simulink model "tennode_3"  (R2018b)
settings: Solver=ode3  StartTime=0.0  StopTime=5  FixedStep=Ts  RelTol=1e-3
values from neighbouring files (symbols this model uses):
  BESS_mode = 0    [load_vars.m]
  line1 = line1_length*R1    (= 0.01273)    [load_vars.m]
  line10 = line10_length*R1    (= 0.01273)    [load_vars.m]
  LINE10_en = 1    [load_vars.m]
  line11 = line11_length*R1    (= 0.01273)    [load_vars.m]
  LINE11_en = 1    [load_vars.m]
  line12 = line12_length*R1    (= 0.02546)    [load_vars.m]
  LINE12_en = 1    [load_vars.m]
  line13 = line13_length*R1    (= 0.015276)    [load_vars.m]
  LINE13_en = 1    [load_vars.m]
  line14 = line14_length*R1    (= 0.019095)    [load_vars.m]
  LINE14_en = 1    [load_vars.m]
  line15 = line15_length*R1    (= 0.014003)    [load_vars.m]
  LINE15_en = 1    [load_vars.m]
  line16 = line16_length*R1    (= 0.034371)    [load_vars.m]
  LINE16_en = 1    [load_vars.m]
  line17 = line17_length*R1    (= 0.017822)    [load_vars.m]
  LINE17_en = 1    [load_vars.m]
  LINE1_en = 1    [load_vars.m]
  line2 = line2_length*R1    (= 0.02546)    [load_vars.m]
  LINE2_en = 1    [load_vars.m]
  line3 = line3_length*R1    (= 0.015276)    [load_vars.m]
  LINE3_en = 1    [load_vars.m]
  line4 = line4_length*R1    (= 0.019095)    [load_vars.m]
  LINE4_en = 1    [load_vars.m]
  line5 = line5_length*R1    (= 0.014003)    [load_vars.m]
  LINE5_en = 1    [load_vars.m]
  line6 = line6_length*R1    (= 0.01273)    [load_vars.m]
  LINE6_en = 1    [load_vars.m]
  line7 = line7_length*R1    (= 0.03819)    [load_vars.m]
  LINE7_en = 1    [load_vars.m]
  line8 = line8_length*R1    (= 0.01273)    [load_vars.m]
  LINE8_en = 1    [load_vars.m]
  line9 = line9_length*R1    (= 0.01273)    [load_vars.m]
  LINE9_en = 1    [load_vars.m]
  t_contingency = 1    [load_vars.m]
  Ts = 0.0001    [load_vars.m]
  uDemand1 = 20e3    (= 20000)    [load_vars.m]
  uDemand10 = 20e3    (= 20000)    [load_vars.m]
  uDemand2 = 20e3    (= 20000)    [load_vars.m]
  uDemand3 = 20e3    (= 20000)    [load_vars.m]
  uDemand4 = 20e3    (= 20000)    [load_vars.m]
  uDemand5 = 20e3    (= 20000)    [load_vars.m]
  uDemand6 = 20e3    (= 20000)    [load_vars.m]
  uDemand7 = 20e3    (= 20000)    [load_vars.m]
  uDemand8 = 20e3    (= 20000)    [load_vars.m]
  uDemand9 = 20e3    (= 20000)    [load_vars.m]
undefined symbols (not defined in the file or in its folder): DER10_BESS_en, DER1_BESS_en, DER2_BESS_en, DER3_BESS_en, DER4_BESS_en, DER5_BESS_en, DER6_BESS_en, DER7_BESS_en, DER8_BESS_en, DER9_BESS_en, DR_capacity_1, DR_capacity_10, DR_capacity_2, DR_capacity_3, DR_capacity_4, DR_capacity_5, DR_capacity_6, DR_capacity_7, DR_capacity_8, DR_capacity_9, P_set1, P_set10, P_set2, P_set3, P_set4, P_set5, P_set6, P_set7, P_set8, P_set9, PV_capacity_1, PV_capacity_10, PV_capacity_2, PV_capacity_3, PV_capacity_4, PV_capacity_5, PV_capacity_6, PV_capacity_7, PV_capacity_8, PV_capacity_9, PV_en_1, PV_en_10, PV_en_2, PV_en_3, PV_en_4, PV_en_5, PV_en_6, PV_en_7, PV_en_8, PV_en_9
libraries: powerlib x232, simulink x66, powerlib_meascontrol x23, sps_avr x1, spsDieselMotorModel x1
(part 6 of 7)

== system tennode_3/DER_Site_3/DER3_BESS/Stored Energy Calculation (%) ==
  Pin : Inport
  Qin : Inport  Port=2
  Charge : Gain  Gain=Efficiency/100
  Compare To Zero : simulink/Logic and Bit Operations/Compare To Zero  relop=<=  OutDataTypeStr=boolean
  Constant : Constant  Value=kWh_Rated
  Discharge : Gain  Gain=1/(Efficiency/100)
  Divide : Product  Inputs=*/
  Gain3 : Gain  Gain=1/3600/1e3
  Gain5 : Gain  Gain=-1
  Integrator : Integrator  InitialCondition=(Initial_kWh_pc/100)*kWh_Rated*3600*1e3
  Math Function1 : Math  Operator=square  SaturateOnIntegerOverflow=on
  Math Function2 : Math  Operator=square  SaturateOnIntegerOverflow=on
  Product : Product
  Sign : Signum
  Sqrt : Sqrt  SaturateOnIntegerOverflow=on
  Sum : Sum  Inputs=|++
  Switch1 : Switch  Criteria=u2 ~= 0
  Transfer Fcn : TransferFcn  Denominator=[1 1]
  to % : Gain  Gain=100
  SE% : Outport
  wires:
  Integrator/1 -> Gain3/1
  Compare To Zero/1 -> Switch1/2
  Divide/1 -> to %/1
  Charge/1 -> Switch1/1
  Constant/1 -> Divide/2
  Gain3/1 -> Divide/1
  Switch1/1 -> Gain5/1
  Transfer Fcn/1 -> Compare To Zero/1
  to %/1 -> SE%/1
  Gain5/1 -> Integrator/1
  Discharge/1 -> Switch1/3
  Product/1 -> Charge/1, Discharge/1, Transfer Fcn/1
  Pin/1 -> Sign/1, Math Function1/1
  Qin/1 -> Math Function2/1
  Math Function1/1 -> Sum/1
  Math Function2/1 -> Sum/2
  Sum/1 -> Sqrt/1
  Sqrt/1 -> Product/2
  Sign/1 -> Product/1

== system tennode_3/DER_Site_3/Site Load/Dynamic Load Control ==
  P0 : Inport
  Fcn : Fcn  Expr=sqrt(1/u(1)-1)
  Mux : Mux  Inputs=2
  Product : Product
  Summer1 : Constant  Value=PF
  PQ : Outport
  wires:
  Summer1/1 -> Fcn/1
  Fcn/1 -> Product/2
  P0/1 -> Product/1, Mux/1
  Mux/1 -> PQ/1
  Product/1 -> Mux/2  "Qo"

== system tennode_3/DER_Site_4/DER3_BESS1/Charge Limits ==
  SOC (%) : Inport
  Pin : Inport  Port=2
  Qin : Inport  Port=3
  Overcharge Check : Subsystem
  Undercharge Check : Subsystem
  Pbatt : Outport
  Qbatt : Outport  Port=2
  wires:
  Overcharge Check/2(Qout) -> Undercharge Check/3(Qin)
  Undercharge Check/1(Pout) -> Pbatt/1  "Pbatt"
  Qin/1 -> Overcharge Check/3(Qin)
  Overcharge Check/1(Pout) -> Undercharge Check/2(Pin)
  Pin/1 -> Overcharge Check/2(Pin)
  Undercharge Check/2(Qout) -> Qbatt/1
  SOC (%)/1 -> Undercharge Check/1(SOC (%)), Overcharge Check/1(SOC (%))

== system tennode_3/DER_Site_4/DER3_BESS1/Disable PQ Source if VF Control ==
  Pdes : Inport
  Mode : Inport  Port=2
  Qdes : Inport  Port=3
  Constant : Constant  Value=0
  Constant1 : Constant  Value=0
  Switch2 : Switch  Criteria=u2 > Threshold
  Switch3 : Switch  Criteria=u2 > Threshold
  Pbatt : Outport
  Qbatt : Outport  Port=2
  wires:
  Qdes/1 -> Switch3/1
  Constant/1 -> Switch2/3
  Switch3/1 -> Qbatt/1
  Constant1/1 -> Switch3/3
  Switch2/1 -> Pbatt/1
  Pdes/1 -> Switch2/1
  Mode/1 -> Switch2/2, Switch3/2

== system tennode_3/DER_Site_4/DER3_BESS1/Power Measures ==
  EMT : Subsystem  VariantControl=EMT
  Phasor : Subsystem  VariantControl=Phasor
  A : PMIOPort  Side=Left
  a : PMIOPort  Port=2  Side=Right
  B : PMIOPort  Port=3  Side=Left
  b : PMIOPort  Port=4  Side=Right
  C : PMIOPort  Port=5  Side=Left
  c : PMIOPort  Port=6  Side=Right
  P : Outport
  Q : Outport  Port=2

== system tennode_3/DER_Site_4/DER3_BESS1/Reactive Power Capability ==
  Pin : Inport
  Qin : Inport  Port=2
  Constant : Constant  Value=Pnom
  Math Function : Math  Operator=square  SaturateOnIntegerOverflow=on
  Math Function1 : Math  Operator=square  SaturateOnIntegerOverflow=on
  Saturation Dynamic : simulink/Discontinuities/Saturation Dynamic  OutMin=[]  OutMax=[]  OutDataTypeStr=Inherit: Same as second input  OutDataType=fixdt(1, 16)  OutScaling=2^-10  DoSatur=off
  Sqrt : Sqrt  SaturateOnIntegerOverflow=on
  Sum : Sum  Inputs=-+|
  Unary Minus : UnaryMinus
  Qout : Outport
  wires:
  Qin/1 -> Saturation Dynamic/2
  Pin/1 -> Math Function1/1
  Saturation Dynamic/1 -> Qout/1
  Unary Minus/1 -> Saturation Dynamic/3
  Sum/1 -> Sqrt/1
  Constant/1 -> Math Function/1
  Math Function/1 -> Sum/2
  Math Function1/1 -> Sum/1
  Sqrt/1 -> Unary Minus/1, Saturation Dynamic/1

== system tennode_3/DER_Site_4/DER3_BESS1/Stored Energy Calculation (%) ==
  Pin : Inport
  Qin : Inport  Port=2
  Charge : Gain  Gain=Efficiency/100
  Compare To Zero : simulink/Logic and Bit Operations/Compare To Zero  relop=<=  OutDataTypeStr=boolean
  Constant : Constant  Value=kWh_Rated
  Discharge : Gain  Gain=1/(Efficiency/100)
  Divide : Product  Inputs=*/
  Gain3 : Gain  Gain=1/3600/1e3
  Gain5 : Gain  Gain=-1
  Integrator : Integrator  InitialCondition=(Initial_kWh_pc/100)*kWh_Rated*3600*1e3
  Math Function1 : Math  Operator=square  SaturateOnIntegerOverflow=on
  Math Function2 : Math  Operator=square  SaturateOnIntegerOverflow=on
  Product : Product
  Sign : Signum
  Sqrt : Sqrt  SaturateOnIntegerOverflow=on
  Sum : Sum  Inputs=|++
  Switch1 : Switch  Criteria=u2 ~= 0
  Transfer Fcn : TransferFcn  Denominator=[1 1]
  to % : Gain  Gain=100
  SE% : Outport
  wires:
  Integrator/1 -> Gain3/1
  Compare To Zero/1 -> Switch1/2
  Divide/1 -> to %/1
  Charge/1 -> Switch1/1
  Constant/1 -> Divide/2
  Gain3/1 -> Divide/1
  Switch1/1 -> Gain5/1
  Transfer Fcn/1 -> Compare To Zero/1
  to %/1 -> SE%/1
  Gain5/1 -> Integrator/1
  Discharge/1 -> Switch1/3
  Product/1 -> Charge/1, Discharge/1, Transfer Fcn/1
  Pin/1 -> Sign/1, Math Function1/1
  Qin/1 -> Math Function2/1
  Math Function1/1 -> Sum/1
  Math Function2/1 -> Sum/2
  Sum/1 -> Sqrt/1
  Sqrt/1 -> Product/2
  Sign/1 -> Product/1

== system tennode_3/DER_Site_4/Site Load/Dynamic Load Control ==
  P0 : Inport
  Fcn : Fcn  Expr=sqrt(1/u(1)-1)
  Mux : Mux  Inputs=2
  Product : Product
  Summer1 : Constant  Value=PF
  PQ : Outport
  wires:
  Summer1/1 -> Fcn/1
  Fcn/1 -> Product/2
  P0/1 -> Product/1, Mux/1
  Mux/1 -> PQ/1
  Product/1 -> Mux/2  "Qo"

== system tennode_3/DER_Site_5/DER3_BESS1/Charge Limits ==
  SOC (%) : Inport
  Pin : Inport  Port=2
  Qin : Inport  Port=3
  Overcharge Check : Subsystem
  Undercharge Check : Subsystem
  Pbatt : Outport
  Qbatt : Outport  Port=2
  wires:
  Overcharge Check/2(Qout) -> Undercharge Check/3(Qin)
  Undercharge Check/1(Pout) -> Pbatt/1  "Pbatt"
  Qin/1 -> Overcharge Check/3(Qin)
  Overcharge Check/1(Pout) -> Undercharge Check/2(Pin)
  Pin/1 -> Overcharge Check/2(Pin)
  Undercharge Check/2(Qout) -> Qbatt/1
  SOC (%)/1 -> Undercharge Check/1(SOC (%)), Overcharge Check/1(SOC (%))

== system tennode_3/DER_Site_5/DER3_BESS1/Disable PQ Source if VF Control ==
  Pdes : Inport
  Mode : Inport  Port=2
  Qdes : Inport  Port=3
  Constant : Constant  Value=0
  Constant1 : Constant  Value=0
  Switch2 : Switch  Criteria=u2 > Threshold
  Switch3 : Switch  Criteria=u2 > Threshold
  Pbatt : Outport
  Qbatt : Outport  Port=2
  wires:
  Qdes/1 -> Switch3/1
  Constant/1 -> Switch2/3
  Switch3/1 -> Qbatt/1
  Constant1/1 -> Switch3/3
  Switch2/1 -> Pbatt/1
  Pdes/1 -> Switch2/1
  Mode/1 -> Switch2/2, Switch3/2

== system tennode_3/DER_Site_5/DER3_BESS1/Power Measures ==
  EMT : Subsystem  VariantControl=EMT
  Phasor : Subsystem  VariantControl=Phasor
  A : PMIOPort  Side=Left
  a : PMIOPort  Port=2  Side=Right
  B : PMIOPort  Port=3  Side=Left
  b : PMIOPort  Port=4  Side=Right
  C : PMIOPort  Port=5  Side=Left
  c : PMIOPort  Port=6  Side=Right
  P : Outport
  Q : Outport  Port=2

== system tennode_3/DER_Site_5/DER3_BESS1/Reactive Power Capability ==
  Pin : Inport
  Qin : Inport  Port=2
  Constant : Constant  Value=Pnom
  Math Function : Math  Operator=square  SaturateOnIntegerOverflow=on
  Math Function1 : Math  Operator=square  SaturateOnIntegerOverflow=on
  Saturation Dynamic : simulink/Discontinuities/Saturation Dynamic  OutMin=[]  OutMax=[]  OutDataTypeStr=Inherit: Same as second input  OutDataType=fixdt(1, 16)  OutScaling=2^-10  DoSatur=off
  Sqrt : Sqrt  SaturateOnIntegerOverflow=on
  Sum : Sum  Inputs=-+|
  Unary Minus : UnaryMinus
  Qout : Outport
  wires:
  Qin/1 -> Saturation Dynamic/2
  Pin/1 -> Math Function1/1
  Saturation Dynamic/1 -> Qout/1
  Unary Minus/1 -> Saturation Dynamic/3
  Sum/1 -> Sqrt/1
  Constant/1 -> Math Function/1
  Math Function/1 -> Sum/2
  Math Function1/1 -> Sum/1
  Sqrt/1 -> Unary Minus/1, Saturation Dynamic/1

== system tennode_3/DER_Site_5/DER3_BESS1/Stored Energy Calculation (%) ==
  Pin : Inport
  Qin : Inport  Port=2
  Charge : Gain  Gain=Efficiency/100
  Compare To Zero : simulink/Logic and Bit Operations/Compare To Zero  relop=<=  OutDataTypeStr=boolean
  Constant : Constant  Value=kWh_Rated
  Discharge : Gain  Gain=1/(Efficiency/100)
  Divide : Product  Inputs=*/
  Gain3 : Gain  Gain=1/3600/1e3
  Gain5 : Gain  Gain=-1
  Integrator : Integrator  InitialCondition=(Initial_kWh_pc/100)*kWh_Rated*3600*1e3
  Math Function1 : Math  Operator=square  SaturateOnIntegerOverflow=on
  Math Function2 : Math  Operator=square  SaturateOnIntegerOverflow=on
  Product : Product
  Sign : Signum
  Sqrt : Sqrt  SaturateOnIntegerOverflow=on
  Sum : Sum  Inputs=|++
  Switch1 : Switch  Criteria=u2 ~= 0
  Transfer Fcn : TransferFcn  Denominator=[1 1]
  to % : Gain  Gain=100
  SE% : Outport
  wires:
  Integrator/1 -> Gain3/1
  Compare To Zero/1 -> Switch1/2
  Divide/1 -> to %/1
  Charge/1 -> Switch1/1
  Constant/1 -> Divide/2
  Gain3/1 -> Divide/1
  Switch1/1 -> Gain5/1
  Transfer Fcn/1 -> Compare To Zero/1
  to %/1 -> SE%/1
  Gain5/1 -> Integrator/1
  Discharge/1 -> Switch1/3
  Product/1 -> Charge/1, Discharge/1, Transfer Fcn/1
  Pin/1 -> Sign/1, Math Function1/1
  Qin/1 -> Math Function2/1
  Math Function1/1 -> Sum/1
  Math Function2/1 -> Sum/2
  Sum/1 -> Sqrt/1
  Sqrt/1 -> Product/2
  Sign/1 -> Product/1

== system tennode_3/DER_Site_5/Site Load/Dynamic Load Control ==
  P0 : Inport
  Fcn : Fcn  Expr=sqrt(1/u(1)-1)
  Mux : Mux  Inputs=2
  Product : Product
  Summer1 : Constant  Value=PF
  PQ : Outport
  wires:
  Summer1/1 -> Fcn/1
  Fcn/1 -> Product/2
  P0/1 -> Product/1, Mux/1
  Mux/1 -> PQ/1
  Product/1 -> Mux/2  "Qo"

== system tennode_3/DER_Site_6/DER6_BESS/Charge Limits ==
  SOC (%) : Inport
  Pin : Inport  Port=2
  Qin : Inport  Port=3
  Overcharge Check : Subsystem
  Undercharge Check : Subsystem
  Pbatt : Outport
  Qbatt : Outport  Port=2
  wires:
  Overcharge Check/2(Qout) -> Undercharge Check/3(Qin)
  Undercharge Check/1(Pout) -> Pbatt/1  "Pbatt"
  Qin/1 -> Overcharge Check/3(Qin)
  Overcharge Check/1(Pout) -> Undercharge Check/2(Pin)
  Pin/1 -> Overcharge Check/2(Pin)
  Undercharge Check/2(Qout) -> Qbatt/1
  SOC (%)/1 -> Undercharge Check/1(SOC (%)), Overcharge Check/1(SOC (%))

== system tennode_3/DER_Site_6/DER6_BESS/Disable PQ Source if VF Control ==
  Pdes : Inport
  Mode : Inport  Port=2
  Qdes : Inport  Port=3
  Constant : Constant  Value=0
  Constant1 : Constant  Value=0
  Switch2 : Switch  Criteria=u2 > Threshold
  Switch3 : Switch  Criteria=u2 > Threshold
  Pbatt : Outport
  Qbatt : Outport  Port=2
  wires:
  Qdes/1 -> Switch3/1
  Constant/1 -> Switch2/3
  Switch3/1 -> Qbatt/1
  Constant1/1 -> Switch3/3
  Switch2/1 -> Pbatt/1
  Pdes/1 -> Switch2/1
  Mode/1 -> Switch2/2, Switch3/2

== system tennode_3/DER_Site_6/DER6_BESS/Power Measures ==
  EMT : Subsystem  VariantControl=EMT
  Phasor : Subsystem  VariantControl=Phasor
  A : PMIOPort  Side=Left
  a : PMIOPort  Port=2  Side=Right
  B : PMIOPort  Port=3  Side=Left
  b : PMIOPort  Port=4  Side=Right
  C : PMIOPort  Port=5  Side=Left
  c : PMIOPort  Port=6  Side=Right
  P : Outport
  Q : Outport  Port=2

== system tennode_3/DER_Site_6/DER6_BESS/Reactive Power Capability ==
  Pin : Inport
  Qin : Inport  Port=2
  Constant : Constant  Value=Pnom
  Math Function : Math  Operator=square  SaturateOnIntegerOverflow=on
  Math Function1 : Math  Operator=square  SaturateOnIntegerOverflow=on
  Saturation Dynamic : simulink/Discontinuities/Saturation Dynamic  OutMin=[]  OutMax=[]  OutDataTypeStr=Inherit: Same as second input  OutDataType=fixdt(1, 16)  OutScaling=2^-10  DoSatur=off
  Sqrt : Sqrt  SaturateOnIntegerOverflow=on
  Sum : Sum  Inputs=-+|
  Unary Minus : UnaryMinus
  Qout : Outport
  wires:
  Qin/1 -> Saturation Dynamic/2
  Pin/1 -> Math Function1/1
  Saturation Dynamic/1 -> Qout/1
  Unary Minus/1 -> Saturation Dynamic/3
  Sum/1 -> Sqrt/1
  Constant/1 -> Math Function/1
  Math Function/1 -> Sum/2
  Math Function1/1 -> Sum/1
  Sqrt/1 -> Unary Minus/1, Saturation Dynamic/1

== system tennode_3/DER_Site_6/DER6_BESS/Stored Energy Calculation (%) ==
  Pin : Inport
  Qin : Inport  Port=2
  Charge : Gain  Gain=Efficiency/100
  Compare To Zero : simulink/Logic and Bit Operations/Compare To Zero  relop=<=  OutDataTypeStr=boolean
  Constant : Constant  Value=kWh_Rated
  Discharge : Gain  Gain=1/(Efficiency/100)
  Divide : Product  Inputs=*/
  Gain3 : Gain  Gain=1/3600/1e3
  Gain5 : Gain  Gain=-1
  Integrator : Integrator  InitialCondition=(Initial_kWh_pc/100)*kWh_Rated*3600*1e3
  Math Function1 : Math  Operator=square  SaturateOnIntegerOverflow=on
  Math Function2 : Math  Operator=square  SaturateOnIntegerOverflow=on
  Product : Product
  Sign : Signum
  Sqrt : Sqrt  SaturateOnIntegerOverflow=on
  Sum : Sum  Inputs=|++
  Switch1 : Switch  Criteria=u2 ~= 0
  Transfer Fcn : TransferFcn  Denominator=[1 1]
  to % : Gain  Gain=100
  SE% : Outport
  wires:
  Integrator/1 -> Gain3/1
  Compare To Zero/1 -> Switch1/2
  Divide/1 -> to %/1
  Charge/1 -> Switch1/1
  Constant/1 -> Divide/2
  Gain3/1 -> Divide/1
  Switch1/1 -> Gain5/1
  Transfer Fcn/1 -> Compare To Zero/1
  to %/1 -> SE%/1
  Gain5/1 -> Integrator/1
  Discharge/1 -> Switch1/3
  Product/1 -> Charge/1, Discharge/1, Transfer Fcn/1
  Pin/1 -> Sign/1, Math Function1/1
  Qin/1 -> Math Function2/1
  Math Function1/1 -> Sum/1
  Math Function2/1 -> Sum/2
  Sum/1 -> Sqrt/1
  Sqrt/1 -> Product/2
  Sign/1 -> Product/1

== system tennode_3/DER_Site_6/Site Load/Dynamic Load Control ==
  P0 : Inport
  Fcn : Fcn  Expr=sqrt(1/u(1)-1)
  Mux : Mux  Inputs=2
  Product : Product
  Summer1 : Constant  Value=PF
  PQ : Outport
  wires:
  Summer1/1 -> Fcn/1
  Fcn/1 -> Product/2
  P0/1 -> Product/1, Mux/1
  Mux/1 -> PQ/1
  Product/1 -> Mux/2  "Qo"

== system tennode_3/DER_Site_7/DER7_BESS/Charge Limits ==
  SOC (%) : Inport
  Pin : Inport  Port=2
  Qin : Inport  Port=3
  Overcharge Check : Subsystem
  Undercharge Check : Subsystem
  Pbatt : Outport
  Qbatt : Outport  Port=2
  wires:
  Overcharge Check/2(Qout) -> Undercharge Check/3(Qin)
  Undercharge Check/1(Pout) -> Pbatt/1  "Pbatt"
  Qin/1 -> Overcharge Check/3(Qin)
  Overcharge Check/1(Pout) -> Undercharge Check/2(Pin)
  Pin/1 -> Overcharge Check/2(Pin)
  Undercharge Check/2(Qout) -> Qbatt/1
  SOC (%)/1 -> Undercharge Check/1(SOC (%)), Overcharge Check/1(SOC (%))

== system tennode_3/DER_Site_7/DER7_BESS/Disable PQ Source if VF Control ==
  Pdes : Inport
  Mode : Inport  Port=2
  Qdes : Inport  Port=3
  Constant : Constant  Value=0
  Constant1 : Constant  Value=0
  Switch2 : Switch  Criteria=u2 > Threshold
  Switch3 : Switch  Criteria=u2 > Threshold
  Pbatt : Outport
  Qbatt : Outport  Port=2
  wires:
  Qdes/1 -> Switch3/1
  Constant/1 -> Switch2/3
  Switch3/1 -> Qbatt/1
  Constant1/1 -> Switch3/3
  Switch2/1 -> Pbatt/1
  Pdes/1 -> Switch2/1
  Mode/1 -> Switch2/2, Switch3/2

== system tennode_3/DER_Site_7/DER7_BESS/Power Measures ==
  EMT : Subsystem  VariantControl=EMT
  Phasor : Subsystem  VariantControl=Phasor
  A : PMIOPort  Side=Left
  a : PMIOPort  Port=2  Side=Right
  B : PMIOPort  Port=3  Side=Left
  b : PMIOPort  Port=4  Side=Right
  C : PMIOPort  Port=5  Side=Left
  c : PMIOPort  Port=6  Side=Right
  P : Outport
  Q : Outport  Port=2

== system tennode_3/DER_Site_7/DER7_BESS/Reactive Power Capability ==
  Pin : Inport
  Qin : Inport  Port=2
  Constant : Constant  Value=Pnom
  Math Function : Math  Operator=square  SaturateOnIntegerOverflow=on
  Math Function1 : Math  Operator=square  SaturateOnIntegerOverflow=on
  Saturation Dynamic : simulink/Discontinuities/Saturation Dynamic  OutMin=[]  OutMax=[]  OutDataTypeStr=Inherit: Same as second input  OutDataType=fixdt(1, 16)  OutScaling=2^-10  DoSatur=off
  Sqrt : Sqrt  SaturateOnIntegerOverflow=on
  Sum : Sum  Inputs=-+|
  Unary Minus : UnaryMinus
  Qout : Outport
  wires:
  Qin/1 -> Saturation Dynamic/2
  Pin/1 -> Math Function1/1
  Saturation Dynamic/1 -> Qout/1
  Unary Minus/1 -> Saturation Dynamic/3
  Sum/1 -> Sqrt/1
  Constant/1 -> Math Function/1
  Math Function/1 -> Sum/2
  Math Function1/1 -> Sum/1
  Sqrt/1 -> Unary Minus/1, Saturation Dynamic/1

== system tennode_3/DER_Site_7/DER7_BESS/Stored Energy Calculation (%) ==
  Pin : Inport
  Qin : Inport  Port=2
  Charge : Gain  Gain=Efficiency/100
  Compare To Zero : simulink/Logic and Bit Operations/Compare To Zero  relop=<=  OutDataTypeStr=boolean
  Constant : Constant  Value=kWh_Rated
  Discharge : Gain  Gain=1/(Efficiency/100)
  Divide : Product  Inputs=*/
  Gain3 : Gain  Gain=1/3600/1e3
  Gain5 : Gain  Gain=-1
  Integrator : Integrator  InitialCondition=(Initial_kWh_pc/100)*kWh_Rated*3600*1e3
  Math Function1 : Math  Operator=square  SaturateOnIntegerOverflow=on
  Math Function2 : Math  Operator=square  SaturateOnIntegerOverflow=on
  Product : Product
  Sign : Signum
  Sqrt : Sqrt  SaturateOnIntegerOverflow=on
  Sum : Sum  Inputs=|++
  Switch1 : Switch  Criteria=u2 ~= 0
  Transfer Fcn : TransferFcn  Denominator=[1 1]
  to % : Gain  Gain=100
  SE% : Outport
  wires:
  Integrator/1 -> Gain3/1
  Compare To Zero/1 -> Switch1/2
  Divide/1 -> to %/1
  Charge/1 -> Switch1/1
  Constant/1 -> Divide/2
  Gain3/1 -> Divide/1
  Switch1/1 -> Gain5/1
  Transfer Fcn/1 -> Compare To Zero/1
  to %/1 -> SE%/1
  Gain5/1 -> Integrator/1
  Discharge/1 -> Switch1/3
  Product/1 -> Charge/1, Discharge/1, Transfer Fcn/1
  Pin/1 -> Sign/1, Math Function1/1
  Qin/1 -> Math Function2/1
  Math Function1/1 -> Sum/1
  Math Function2/1 -> Sum/2
  Sum/1 -> Sqrt/1
  Sqrt/1 -> Product/2
  Sign/1 -> Product/1

== system tennode_3/DER_Site_7/Site Load/Dynamic Load Control ==
  P0 : Inport
  Fcn : Fcn  Expr=sqrt(1/u(1)-1)
  Mux : Mux  Inputs=2
  Product : Product
  Summer1 : Constant  Value=PF
  PQ : Outport
  wires:
  Summer1/1 -> Fcn/1
  Fcn/1 -> Product/2
  P0/1 -> Product/1, Mux/1
  Mux/1 -> PQ/1
  Product/1 -> Mux/2  "Qo"

== system tennode_3/DER_Site_8/DER8_BESS/Charge Limits ==
  SOC (%) : Inport
  Pin : Inport  Port=2
  Qin : Inport  Port=3
  Overcharge Check : Subsystem
  Undercharge Check : Subsystem
  Pbatt : Outport
  Qbatt : Outport  Port=2
  wires:
  Overcharge Check/2(Qout) -> Undercharge Check/3(Qin)
  Undercharge Check/1(Pout) -> Pbatt/1  "Pbatt"
  Qin/1 -> Overcharge Check/3(Qin)
  Overcharge Check/1(Pout) -> Undercharge Check/2(Pin)
  Pin/1 -> Overcharge Check/2(Pin)
  Undercharge Check/2(Qout) -> Qbatt/1
  SOC (%)/1 -> Undercharge Check/1(SOC (%)), Overcharge Check/1(SOC (%))

== system tennode_3/DER_Site_8/DER8_BESS/Disable PQ Source if VF Control ==
  Pdes : Inport
  Mode : Inport  Port=2
  Qdes : Inport  Port=3
  Constant : Constant  Value=0
  Constant1 : Constant  Value=0
  Switch2 : Switch  Criteria=u2 > Threshold
  Switch3 : Switch  Criteria=u2 > Threshold
  Pbatt : Outport
  Qbatt : Outport  Port=2
  wires:
  Qdes/1 -> Switch3/1
  Constant/1 -> Switch2/3
  Switch3/1 -> Qbatt/1
  Constant1/1 -> Switch3/3
  Switch2/1 -> Pbatt/1
  Pdes/1 -> Switch2/1
  Mode/1 -> Switch2/2, Switch3/2

== system tennode_3/DER_Site_8/DER8_BESS/Power Measures ==
  EMT : Subsystem  VariantControl=EMT
  Phasor : Subsystem  VariantControl=Phasor
  A : PMIOPort  Side=Left
  a : PMIOPort  Port=2  Side=Right
  B : PMIOPort  Port=3  Side=Left
  b : PMIOPort  Port=4  Side=Right
  C : PMIOPort  Port=5  Side=Left
  c : PMIOPort  Port=6  Side=Right
  P : Outport
  Q : Outport  Port=2

== system tennode_3/DER_Site_8/DER8_BESS/Reactive Power Capability ==
  Pin : Inport
  Qin : Inport  Port=2
  Constant : Constant  Value=Pnom
  Math Function : Math  Operator=square  SaturateOnIntegerOverflow=on
  Math Function1 : Math  Operator=square  SaturateOnIntegerOverflow=on
  Saturation Dynamic : simulink/Discontinuities/Saturation Dynamic  OutMin=[]  OutMax=[]  OutDataTypeStr=Inherit: Same as second input  OutDataType=fixdt(1, 16)  OutScaling=2^-10  DoSatur=off
  Sqrt : Sqrt  SaturateOnIntegerOverflow=on
  Sum : Sum  Inputs=-+|
  Unary Minus : UnaryMinus
  Qout : Outport
  wires:
  Qin/1 -> Saturation Dynamic/2
  Pin/1 -> Math Function1/1
  Saturation Dynamic/1 -> Qout/1
  Unary Minus/1 -> Saturation Dynamic/3
  Sum/1 -> Sqrt/1
  Constant/1 -> Math Function/1
  Math Function/1 -> Sum/2
  Math Function1/1 -> Sum/1
  Sqrt/1 -> Unary Minus/1, Saturation Dynamic/1

== system tennode_3/DER_Site_8/DER8_BESS/Stored Energy Calculation (%) ==
  Pin : Inport
  Qin : Inport  Port=2
  Charge : Gain  Gain=Efficiency/100
  Compare To Zero : simulink/Logic and Bit Operations/Compare To Zero  relop=<=  OutDataTypeStr=boolean
  Constant : Constant  Value=kWh_Rated
  Discharge : Gain  Gain=1/(Efficiency/100)
  Divide : Product  Inputs=*/
  Gain3 : Gain  Gain=1/3600/1e3
  Gain5 : Gain  Gain=-1
  Integrator : Integrator  InitialCondition=(Initial_kWh_pc/100)*kWh_Rated*3600*1e3
  Math Function1 : Math  Operator=square  SaturateOnIntegerOverflow=on
  Math Function2 : Math  Operator=square  SaturateOnIntegerOverflow=on
  Product : Product
  Sign : Signum
  Sqrt : Sqrt  SaturateOnIntegerOverflow=on
  Sum : Sum  Inputs=|++
  Switch1 : Switch  Criteria=u2 ~= 0
  Transfer Fcn : TransferFcn  Denominator=[1 1]
  to % : Gain  Gain=100
  SE% : Outport
  wires:
  Integrator/1 -> Gain3/1
  Compare To Zero/1 -> Switch1/2
  Divide/1 -> to %/1
  Charge/1 -> Switch1/1
  Constant/1 -> Divide/2
  Gain3/1 -> Divide/1
  Switch1/1 -> Gain5/1
  Transfer Fcn/1 -> Compare To Zero/1
  to %/1 -> SE%/1
  Gain5/1 -> Integrator/1
  Discharge/1 -> Switch1/3
  Product/1 -> Charge/1, Discharge/1, Transfer Fcn/1
  Pin/1 -> Sign/1, Math Function1/1
  Qin/1 -> Math Function2/1
  Math Function1/1 -> Sum/1
  Math Function2/1 -> Sum/2
  Sum/1 -> Sqrt/1
  Sqrt/1 -> Product/2
  Sign/1 -> Product/1

== system tennode_3/DER_Site_8/Site Load/Dynamic Load Control ==
  P0 : Inport
  Fcn : Fcn  Expr=sqrt(1/u(1)-1)
  Mux : Mux  Inputs=2
  Product : Product
  Summer1 : Constant  Value=PF
  PQ : Outport
  wires:
  Summer1/1 -> Fcn/1
  Fcn/1 -> Product/2
  P0/1 -> Product/1, Mux/1
  Mux/1 -> PQ/1
  Product/1 -> Mux/2  "Qo"

== system tennode_3/DER_Site_9/DER9_BESS/Charge Limits ==
  SOC (%) : Inport
  Pin : Inport  Port=2
  Qin : Inport  Port=3
  Overcharge Check : Subsystem
  Undercharge Check : Subsystem
  Pbatt : Outport
  Qbatt : Outport  Port=2
  wires:
  Overcharge Check/2(Qout) -> Undercharge Check/3(Qin)
  Undercharge Check/1(Pout) -> Pbatt/1  "Pbatt"
  Qin/1 -> Overcharge Check/3(Qin)
  Overcharge Check/1(Pout) -> Undercharge Check/2(Pin)
  Pin/1 -> Overcharge Check/2(Pin)
  Undercharge Check/2(Qout) -> Qbatt/1
  SOC (%)/1 -> Undercharge Check/1(SOC (%)), Overcharge Check/1(SOC (%))

== system tennode_3/DER_Site_9/DER9_BESS/Disable PQ Source if VF Control ==
  Pdes : Inport
  Mode : Inport  Port=2
  Qdes : Inport  Port=3
  Constant : Constant  Value=0
  Constant1 : Constant  Value=0
  Switch2 : Switch  Criteria=u2 > Threshold
  Switch3 : Switch  Criteria=u2 > Threshold
  Pbatt : Outport
  Qbatt : Outport  Port=2
  wires:
  Qdes/1 -> Switch3/1
  Constant/1 -> Switch2/3
  Switch3/1 -> Qbatt/1
  Constant1/1 -> Switch3/3
  Switch2/1 -> Pbatt/1
  Pdes/1 -> Switch2/1
  Mode/1 -> Switch2/2, Switch3/2

== system tennode_3/DER_Site_9/DER9_BESS/Power Measures ==
  EMT : Subsystem  VariantControl=EMT
  Phasor : Subsystem  VariantControl=Phasor
  A : PMIOPort  Side=Left
  a : PMIOPort  Port=2  Side=Right
  B : PMIOPort  Port=3  Side=Left
  b : PMIOPort  Port=4  Side=Right
  C : PMIOPort  Port=5  Side=Left
  c : PMIOPort  Port=6  Side=Right
  P : Outport
  Q : Outport  Port=2

== system tennode_3/DER_Site_9/DER9_BESS/Reactive Power Capability ==
  Pin : Inport
  Qin : Inport  Port=2
  Constant : Constant  Value=Pnom
  Math Function : Math  Operator=square  SaturateOnIntegerOverflow=on
  Math Function1 : Math  Operator=square  SaturateOnIntegerOverflow=on
  Saturation Dynamic : simulink/Discontinuities/Saturation Dynamic  OutMin=[]  OutMax=[]  OutDataTypeStr=Inherit: Same as second input  OutDataType=fixdt(1, 16)  OutScaling=2^-10  DoSatur=off
  Sqrt : Sqrt  SaturateOnIntegerOverflow=on
  Sum : Sum  Inputs=-+|
  Unary Minus : UnaryMinus
  Qout : Outport
  wires:
  Qin/1 -> Saturation Dynamic/2
  Pin/1 -> Math Function1/1
  Saturation Dynamic/1 -> Qout/1
  Unary Minus/1 -> Saturation Dynamic/3
  Sum/1 -> Sqrt/1
  Constant/1 -> Math Function/1
  Math Function/1 -> Sum/2
  Math Function1/1 -> Sum/1
  Sqrt/1 -> Unary Minus/1, Saturation Dynamic/1

== system tennode_3/DER_Site_9/DER9_BESS/Stored Energy Calculation (%) ==
  Pin : Inport
  Qin : Inport  Port=2
  Charge : Gain  Gain=Efficiency/100
  Compare To Zero : simulink/Logic and Bit Operations/Compare To Zero  relop=<=  OutDataTypeStr=boolean
  Constant : Constant  Value=kWh_Rated
  Discharge : Gain  Gain=1/(Efficiency/100)
  Divide : Product  Inputs=*/
  Gain3 : Gain  Gain=1/3600/1e3
  Gain5 : Gain  Gain=-1
  Integrator : Integrator  InitialCondition=(Initial_kWh_pc/100)*kWh_Rated*3600*1e3
  Math Function1 : Math  Operator=square  SaturateOnIntegerOverflow=on
  Math Function2 : Math  Operator=square  SaturateOnIntegerOverflow=on
  Product : Product
  Sign : Signum
  Sqrt : Sqrt  SaturateOnIntegerOverflow=on
  Sum : Sum  Inputs=|++
  Switch1 : Switch  Criteria=u2 ~= 0
  Transfer Fcn : TransferFcn  Denominator=[1 1]
  to % : Gain  Gain=100
  SE% : Outport
  wires:
  Integrator/1 -> Gain3/1
  Compare To Zero/1 -> Switch1/2
  Divide/1 -> to %/1
  Charge/1 -> Switch1/1
  Constant/1 -> Divide/2
  Gain3/1 -> Divide/1
  Switch1/1 -> Gain5/1
  Transfer Fcn/1 -> Compare To Zero/1
  to %/1 -> SE%/1
  Gain5/1 -> Integrator/1
  Discharge/1 -> Switch1/3
  Product/1 -> Charge/1, Discharge/1, Transfer Fcn/1
  Pin/1 -> Sign/1, Math Function1/1
  Qin/1 -> Math Function2/1
  Math Function1/1 -> Sum/1
  Math Function2/1 -> Sum/2
  Sum/1 -> Sqrt/1
  Sqrt/1 -> Product/2
  Sign/1 -> Product/1

== system tennode_3/DER_Site_9/Site Load/Dynamic Load Control ==
  P0 : Inport
  Fcn : Fcn  Expr=sqrt(1/u(1)-1)
  Mux : Mux  Inputs=2
  Product : Product
  Summer1 : Constant  Value=PF
  PQ : Outport
  wires:
  Summer1/1 -> Fcn/1
  Fcn/1 -> Product/2
  P0/1 -> Product/1, Mux/1
  Mux/1 -> PQ/1
  Product/1 -> Mux/2  "Qo"

== system tennode_3/Frequency Measure/Diesel Generator/Generator Measures ==
  m : Inport
  Bus Selector : BusSelector  OutputSignals="dq0 components.Stator voltage  vq (pu),dq0 components.Stator voltage  vd (pu)"  OutputAsBus=on
  Bus Selector1 : BusSelector  OutputSignals="Mechanical.Rotor speed  wm  (pu),dq0 components.Field current  ifd (pu)"
  Fcn1 : Fcn  Expr=sqrt(u(1)^2 + u(2)^2)
  Ifd : Outport
  Vt : Outport  Port=2
  wm : Outport  Port=3
  wires:
  Bus Selector1/1 -> wm/1  "<Rotor speed  wm  (pu)>"
  m/1 -> Bus Selector1/1, Bus Selector/1
  Fcn1/1 -> Vt/1
  Bus Selector/1 -> Fcn1/1
  Bus Selector1/2 -> Ifd/1  "<Field current  ifd (pu)>"

== system tennode_3/Frequency Measure/Diesel Generator/Selected Measurements ==
  m : Inport
  Bus Creator : BusCreator  Inputs=7
  Bus Selector : BusSelector  OutputSignals="Mechanical.Electrical power  Pe (pu),Mechanical.Rotor speed  wm  (pu),Output active power   Peo (pu),Output reactive power  Qeo (pu)"
  to W : Gain  Gain=Pn
  to W1 : Gain  Gain=Pn
  to W2 : Gain  Gain=Pn
  sm : Outport
  wires:
  to W2/1 -> Bus Creator/7  "Reactive Power (W)"
  to W1/1 -> Bus Creator/6  "Active Power (W)"
  Bus Selector/2 -> Bus Creator/3  "<Rotor speed  wm  (pu)>"
  Bus Creator/1 -> sm/1
  to W/1 -> Bus Creator/1  "Electrical Power (W)"
  Bus Selector/3 -> Bus Creator/4, to W1/1  "<Output active power   Peo (pu)>"
  Bus Selector/1 -> to W/1, Bus Creator/2  "<Electrical power  Pe (pu)>"
  Bus Selector/4 -> Bus Creator/5, to W2/1  "<Output reactive power  Qeo (pu)>"
  m/1 -> Bus Selector/1

== system tennode_3/DER_Site_1/DER_BESS1/Charge Limits/Overcharge Check ==
  SOC (%) : Inport
  Pin : Inport  Port=2
  Qin : Inport  Port=3
  Backlash : Backlash  BacklashWidth=1e-3  InitialOutput=Initial_kWh_pc  ZeroCross=off
  Compare To Constant : simulink/Logic and Bit Operations/Compare To Constant  relop=>  const=UpChrgLim  OutDataTypeStr=boolean
  Compare To Zero : simulink/Logic and Bit Operations/Compare To Zero  relop=<=  OutDataTypeStr=boolean
  Constant : Constant  Value=0
  Constant1 : Constant  Value=0
  Logical Operator : Logic  AllPortsSameDT=off  OutDataTypeStr=boolean
  Switch : Switch  Criteria=u2 ~= 0
  Switch1 : Switch  Criteria=u2 ~= 0
  Pout : Outport
  Qout : Outport  Port=2
  wires:
  Compare To Constant/1 -> Logical Operator/1
  Logical Operator/1 -> Switch1/2, Switch/2
  Constant/1 -> Switch/1
  SOC (%)/1 -> Backlash/1
  Pin/1 -> Compare To Zero/1, Switch/3
  Switch/1 -> Pout/1
  Compare To Zero/1 -> Logical Operator/2
  Qin/1 -> Switch1/3
  Constant1/1 -> Switch1/1
  Switch1/1 -> Qout/1
  Backlash/1 -> Compare To Constant/1

== system tennode_3/DER_Site_1/DER_BESS1/Charge Limits/Undercharge Check ==
  SOC (%) : Inport
  Pin : Inport  Port=2
  Qin : Inport  Port=3
  Backlash : Backlash  BacklashWidth=1e-3  InitialOutput=Initial_kWh_pc  ZeroCross=off
  Compare To Constant1 : simulink/Logic and Bit Operations/Compare To Constant  relop=<  const=LowChrgLim  OutDataTypeStr=boolean
  Compare To Zero : simulink/Logic and Bit Operations/Compare To Zero  relop=>  OutDataTypeStr=boolean
  Constant{,1..3} (4 alike) : Constant  Value=0
  Constant4 : Constant  Value=autoRecharge
  IC : InitialCondition  Value=RechargeSOC
  Logical Operator : Logic  AllPortsSameDT=off  OutDataTypeStr=boolean
  Relay : Relay  OnSwitchValue=RechargeSOC  OffSwitchValue=LowChrgLim  OnOutputValue=0  OffOutputValue=-Precharge/100*Pnom
  Switch{,1..4} (5 alike) : Switch  Criteria=u2 ~= 0
  Pout : Outport
  Qout : Outport  Port=2
  wires:
  Compare To Zero/1 -> Logical Operator/2
  Pin/1 -> Switch/3, Compare To Zero/1
  SOC (%)/1 -> Backlash/1
  Constant/1 -> Switch/1
  Logical Operator/1 -> Switch/2, Switch1/2
  Compare To Constant1/1 -> Logical Operator/1
  Constant1/1 -> Switch1/1
  Qin/1 -> Switch1/3
  Backlash/1 -> IC/1, Compare To Constant1/1
  Switch4/1 -> Switch2/1, Switch2/2, Switch3/2
  IC/1 -> Relay/1
  Switch/1 -> Switch2/3
  Switch2/1 -> Pout/1
  Switch3/1 -> Qout/1
  Switch1/1 -> Switch3/3
  Constant2/1 -> Switch3/1
  Relay/1 -> Switch4/1
  Constant3/1 -> Switch4/3
  Constant4/1 -> Switch4/2

== system tennode_3/DER_Site_1/DER_BESS1/Power Measures/EMT ==
  "Power (3ph, Instantaneous)" : powerlib_meascontrol/Measurements/Power (3ph, Instantaneous)
      settings: SourceProductName=Simscape Electrical
  Three-Phase V-I Measurement : powerlib/Measurements/Three-Phase V-I Measurement  VoltageMeasurement=phase-to-ground  SetLabelV=off  LabelV=Vabc  Vpu=off  VpuLL=off  CurrentMeasurement=yes  SetLabelI=off  LabelI=Iabc  Ipu=off  Pbase=100e6  Vbase=500e3  OutputType=Complex  PhasorSimulation=on  PSBequivalent=0
      settings: SourceProductName=Simscape Electrical
  A : PMIOPort  Side=Left
  a : PMIOPort  Port=2  Side=Right
  B : PMIOPort  Port=3  Side=Left
  b : PMIOPort  Port=4  Side=Right
  C : PMIOPort  Port=5  Side=Left
  c : PMIOPort  Port=6  Side=Right
  P : Outport
  Q : Outport  Port=2
  wires:
  "Power (3ph, Instantaneous)"/2 -> Q/1
  "Power (3ph, Instantaneous)"/1 -> P/1
  Three-Phase V-I Measurement/1 -> "Power (3ph, Instantaneous)"/1
  Three-Phase V-I Measurement/2 -> "Power (3ph, Instantaneous)"/2
  connections:
  C/RConn1 -- Three-Phase V-I Measurement/LConn3
  c/RConn1 -- Three-Phase V-I Measurement/RConn3
  Three-Phase V-I Measurement/LConn2 -- B/RConn1
  A/RConn1 -- Three-Phase V-I Measurement/LConn1
  b/RConn1 -- Three-Phase V-I Measurement/RConn2
  Three-Phase V-I Measurement/RConn1 -- a/RConn1

== system tennode_3/DER_Site_1/DER_BESS1/Power Measures/Phasor ==
  "Power (3ph, Phasor)" : powerlib_meascontrol/Measurements/Power (3ph, Phasor)
      settings: SourceProductName=Simscape Electrical  SourceProductBaseCode=PS
  Three-Phase V-I Measurement : powerlib/Measurements/Three-Phase V-I Measurement  VoltageMeasurement=phase-to-ground  SetLabelV=off  LabelV=Vabc  Vpu=off  VpuLL=off  CurrentMeasurement=yes  SetLabelI=off  LabelI=Iabc  Ipu=off  Pbase=100e6  Vbase=500e3  OutputType=Complex  PhasorSimulation=on  PSBequivalent=0
      settings: SourceProductName=Simscape Electrical
  A : PMIOPort  Side=Left
  a : PMIOPort  Port=2  Side=Right
  B : PMIOPort  Port=3  Side=Left
  b : PMIOPort  Port=4  Side=Right
  C : PMIOPort  Port=5  Side=Left
  c : PMIOPort  Port=6  Side=Right
  P : Outport
  Q : Outport  Port=2
  wires:
  Three-Phase V-I Measurement/2 -> "Power (3ph, Phasor)"/2
  Three-Phase V-I Measurement/1 -> "Power (3ph, Phasor)"/1
  "Power (3ph, Phasor)"/1 -> P/1
  "Power (3ph, Phasor)"/2 -> Q/1
  connections:
  Three-Phase V-I Measurement/RConn1 -- a/RConn1
  b/RConn1 -- Three-Phase V-I Measurement/RConn2
  A/RConn1 -- Three-Phase V-I Measurement/LConn1
  Three-Phase V-I Measurement/LConn2 -- B/RConn1
  c/RConn1 -- Three-Phase V-I Measurement/RConn3
  C/RConn1 -- Three-Phase V-I Measurement/LConn3

== system tennode_3/DER_Site_10/DER10_BESS/Charge Limits/Overcharge Check ==
  SOC (%) : Inport
  Pin : Inport  Port=2
  Qin : Inport  Port=3
  Backlash : Backlash  BacklashWidth=1e-3  InitialOutput=Initial_kWh_pc  ZeroCross=off
  Compare To Constant : simulink/Logic and Bit Operations/Compare To Constant  relop=>  const=UpChrgLim  OutDataTypeStr=boolean
  Compare To Zero : simulink/Logic and Bit Operations/Compare To Zero  relop=<=  OutDataTypeStr=boolean
  Constant : Constant  Value=0
  Constant1 : Constant  Value=0
  Logical Operator : Logic  AllPortsSameDT=off  OutDataTypeStr=boolean
  Switch : Switch  Criteria=u2 ~= 0
  Switch1 : Switch  Criteria=u2 ~= 0
  Pout : Outport
  Qout : Outport  Port=2
  wires:
  Compare To Constant/1 -> Logical Operator/1
  Logical Operator/1 -> Switch1/2, Switch/2
  Constant/1 -> Switch/1
  SOC (%)/1 -> Backlash/1
  Pin/1 -> Compare To Zero/1, Switch/3
  Switch/1 -> Pout/1
  Compare To Zero/1 -> Logical Operator/2
  Qin/1 -> Switch1/3
  Constant1/1 -> Switch1/1
  Switch1/1 -> Qout/1
  Backlash/1 -> Compare To Constant/1

== system tennode_3/DER_Site_10/DER10_BESS/Charge Limits/Undercharge Check ==
  SOC (%) : Inport
  Pin : Inport  Port=2
  Qin : Inport  Port=3
  Backlash : Backlash  BacklashWidth=1e-3  InitialOutput=Initial_kWh_pc  ZeroCross=off
  Compare To Constant1 : simulink/Logic and Bit Operations/Compare To Constant  relop=<  const=LowChrgLim  OutDataTypeStr=boolean
  Compare To Zero : simulink/Logic and Bit Operations/Compare To Zero  relop=>  OutDataTypeStr=boolean
  Constant{,1..3} (4 alike) : Constant  Value=0
  Constant4 : Constant  Value=autoRecharge
  IC : InitialCondition  Value=RechargeSOC
  Logical Operator : Logic  AllPortsSameDT=off  OutDataTypeStr=boolean
  Relay : Relay  OnSwitchValue=RechargeSOC  OffSwitchValue=LowChrgLim  OnOutputValue=0  OffOutputValue=-Precharge/100*Pnom
  Switch{,1..4} (5 alike) : Switch  Criteria=u2 ~= 0
  Pout : Outport
  Qout : Outport  Port=2
  wires:
  Compare To Zero/1 -> Logical Operator/2
  Pin/1 -> Switch/3, Compare To Zero/1
  SOC (%)/1 -> Backlash/1
  Constant/1 -> Switch/1
  Logical Operator/1 -> Switch/2, Switch1/2
  Compare To Constant1/1 -> Logical Operator/1
  Constant1/1 -> Switch1/1
  Qin/1 -> Switch1/3
  Backlash/1 -> IC/1, Compare To Constant1/1
  Switch4/1 -> Switch2/1, Switch2/2, Switch3/2
  IC/1 -> Relay/1
  Switch/1 -> Switch2/3
  Switch2/1 -> Pout/1
  Switch3/1 -> Qout/1
  Switch1/1 -> Switch3/3
  Constant2/1 -> Switch3/1
  Relay/1 -> Switch4/1
  Constant3/1 -> Switch4/3
  Constant4/1 -> Switch4/2

== system tennode_3/DER_Site_10/DER10_BESS/Power Measures/EMT ==
  "Power (3ph, Instantaneous)" : powerlib_meascontrol/Measurements/Power (3ph, Instantaneous)
      settings: SourceProductName=Simscape Electrical
  Three-Phase V-I Measurement : powerlib/Measurements/Three-Phase V-I Measurement  VoltageMeasurement=phase-to-ground  SetLabelV=off  LabelV=Vabc  Vpu=off  VpuLL=off  CurrentMeasurement=yes  SetLabelI=off  LabelI=Iabc  Ipu=off  Pbase=100e6  Vbase=500e3  OutputType=Complex  PhasorSimulation=on  PSBequivalent=0
      settings: SourceProductName=Simscape Electrical
  A : PMIOPort  Side=Left
  a : PMIOPort  Port=2  Side=Right
  B : PMIOPort  Port=3  Side=Left
  b : PMIOPort  Port=4  Side=Right
  C : PMIOPort  Port=5  Side=Left
  c : PMIOPort  Port=6  Side=Right
  P : Outport
  Q : Outport  Port=2
  wires:
  "Power (3ph, Instantaneous)"/2 -> Q/1
  "Power (3ph, Instantaneous)"/1 -> P/1
  Three-Phase V-I Measurement/1 -> "Power (3ph, Instantaneous)"/1
  Three-Phase V-I Measurement/2 -> "Power (3ph, Instantaneous)"/2
  connections:
  C/RConn1 -- Three-Phase V-I Measurement/LConn3
  c/RConn1 -- Three-Phase V-I Measurement/RConn3
  Three-Phase V-I Measurement/LConn2 -- B/RConn1
  A/RConn1 -- Three-Phase V-I Measurement/LConn1
  b/RConn1 -- Three-Phase V-I Measurement/RConn2
  Three-Phase V-I Measurement/RConn1 -- a/RConn1

== system tennode_3/DER_Site_10/DER10_BESS/Power Measures/Phasor ==
  "Power (3ph, Phasor)" : powerlib_meascontrol/Measurements/Power (3ph, Phasor)
      settings: SourceProductName=Simscape Electrical  SourceProductBaseCode=PS
  Three-Phase V-I Measurement : powerlib/Measurements/Three-Phase V-I Measurement  VoltageMeasurement=phase-to-ground  SetLabelV=off  LabelV=Vabc  Vpu=off  VpuLL=off  CurrentMeasurement=yes  SetLabelI=off  LabelI=Iabc  Ipu=off  Pbase=100e6  Vbase=500e3  OutputType=Complex  PhasorSimulation=on  PSBequivalent=0
      settings: SourceProductName=Simscape Electrical
  A : PMIOPort  Side=Left
  a : PMIOPort  Port=2  Side=Right
  B : PMIOPort  Port=3  Side=Left
  b : PMIOPort  Port=4  Side=Right
  C : PMIOPort  Port=5  Side=Left
  c : PMIOPort  Port=6  Side=Right
  P : Outport
  Q : Outport  Port=2
  wires:
  Three-Phase V-I Measurement/2 -> "Power (3ph, Phasor)"/2
  Three-Phase V-I Measurement/1 -> "Power (3ph, Phasor)"/1
  "Power (3ph, Phasor)"/1 -> P/1
  "Power (3ph, Phasor)"/2 -> Q/1
  connections:
  Three-Phase V-I Measurement/RConn1 -- a/RConn1
  b/RConn1 -- Three-Phase V-I Measurement/RConn2
  A/RConn1 -- Three-Phase V-I Measurement/LConn1
  Three-Phase V-I Measurement/LConn2 -- B/RConn1
  c/RConn1 -- Three-Phase V-I Measurement/RConn3
  C/RConn1 -- Three-Phase V-I Measurement/LConn3

== system tennode_3/DER_Site_2/DER2_BESS/Charge Limits/Overcharge Check ==
  SOC (%) : Inport
  Pin : Inport  Port=2
  Qin : Inport  Port=3
  Backlash : Backlash  BacklashWidth=1e-3  InitialOutput=Initial_kWh_pc  ZeroCross=off
  Compare To Constant : simulink/Logic and Bit Operations/Compare To Constant  relop=>  const=UpChrgLim  OutDataTypeStr=boolean
  Compare To Zero : simulink/Logic and Bit Operations/Compare To Zero  relop=<=  OutDataTypeStr=boolean
  Constant : Constant  Value=0
  Constant1 : Constant  Value=0
  Logical Operator : Logic  AllPortsSameDT=off  OutDataTypeStr=boolean
  Switch : Switch  Criteria=u2 ~= 0
  Switch1 : Switch  Criteria=u2 ~= 0
  Pout : Outport
  Qout : Outport  Port=2
  wires:
  Compare To Constant/1 -> Logical Operator/1
  Logical Operator/1 -> Switch1/2, Switch/2
  Constant/1 -> Switch/1
  SOC (%)/1 -> Backlash/1
  Pin/1 -> Compare To Zero/1, Switch/3
  Switch/1 -> Pout/1
  Compare To Zero/1 -> Logical Operator/2
  Qin/1 -> Switch1/3
  Constant1/1 -> Switch1/1
  Switch1/1 -> Qout/1
  Backlash/1 -> Compare To Constant/1

== system tennode_3/DER_Site_2/DER2_BESS/Charge Limits/Undercharge Check ==
  SOC (%) : Inport
  Pin : Inport  Port=2
  Qin : Inport  Port=3
  Backlash : Backlash  BacklashWidth=1e-3  InitialOutput=Initial_kWh_pc  ZeroCross=off
  Compare To Constant1 : simulink/Logic and Bit Operations/Compare To Constant  relop=<  const=LowChrgLim  OutDataTypeStr=boolean
  Compare To Zero : simulink/Logic and Bit Operations/Compare To Zero  relop=>  OutDataTypeStr=boolean
  Constant{,1..3} (4 alike) : Constant  Value=0
  Constant4 : Constant  Value=autoRecharge
  IC : InitialCondition  Value=RechargeSOC
  Logical Operator : Logic  AllPortsSameDT=off  OutDataTypeStr=boolean
  Relay : Relay  OnSwitchValue=RechargeSOC  OffSwitchValue=LowChrgLim  OnOutputValue=0  OffOutputValue=-Precharge/100*Pnom
  Switch{,1..4} (5 alike) : Switch  Criteria=u2 ~= 0
  Pout : Outport
  Qout : Outport  Port=2
  wires:
  Compare To Zero/1 -> Logical Operator/2
  Pin/1 -> Switch/3, Compare To Zero/1
  SOC (%)/1 -> Backlash/1
  Constant/1 -> Switch/1
  Logical Operator/1 -> Switch/2, Switch1/2
  Compare To Constant1/1 -> Logical Operator/1
  Constant1/1 -> Switch1/1
  Qin/1 -> Switch1/3
  Backlash/1 -> IC/1, Compare To Constant1/1
  Switch4/1 -> Switch2/1, Switch2/2, Switch3/2
  IC/1 -> Relay/1
  Switch/1 -> Switch2/3
  Switch2/1 -> Pout/1
  Switch3/1 -> Qout/1
  Switch1/1 -> Switch3/3
  Constant2/1 -> Switch3/1
  Relay/1 -> Switch4/1
  Constant3/1 -> Switch4/3
  Constant4/1 -> Switch4/2

== system tennode_3/DER_Site_2/DER2_BESS/Power Measures/EMT ==
  "Power (3ph, Instantaneous)" : powerlib_meascontrol/Measurements/Power (3ph, Instantaneous)
      settings: SourceProductName=Simscape Electrical
  Three-Phase V-I Measurement : powerlib/Measurements/Three-Phase V-I Measurement  VoltageMeasurement=phase-to-ground  SetLabelV=off  LabelV=Vabc  Vpu=off  VpuLL=off  CurrentMeasurement=yes  SetLabelI=off  LabelI=Iabc  Ipu=off  Pbase=100e6  Vbase=500e3  OutputType=Complex  PhasorSimulation=on  PSBequivalent=0
      settings: SourceProductName=Simscape Electrical
  A : PMIOPort  Side=Left
  a : PMIOPort  Port=2  Side=Right
  B : PMIOPort  Port=3  Side=Left
  b : PMIOPort  Port=4  Side=Right
  C : PMIOPort  Port=5  Side=Left
  c : PMIOPort  Port=6  Side=Right
  P : Outport
  Q : Outport  Port=2
  wires:
  "Power (3ph, Instantaneous)"/2 -> Q/1
  "Power (3ph, Instantaneous)"/1 -> P/1
  Three-Phase V-I Measurement/1 -> "Power (3ph, Instantaneous)"/1
  Three-Phase V-I Measurement/2 -> "Power (3ph, Instantaneous)"/2
  connections:
  C/RConn1 -- Three-Phase V-I Measurement/LConn3
  c/RConn1 -- Three-Phase V-I Measurement/RConn3
  Three-Phase V-I Measurement/LConn2 -- B/RConn1
  A/RConn1 -- Three-Phase V-I Measurement/LConn1
  b/RConn1 -- Three-Phase V-I Measurement/RConn2
  Three-Phase V-I Measurement/RConn1 -- a/RConn1

== system tennode_3/DER_Site_2/DER2_BESS/Power Measures/Phasor ==
  "Power (3ph, Phasor)" : powerlib_meascontrol/Measurements/Power (3ph, Phasor)
      settings: SourceProductName=Simscape Electrical  SourceProductBaseCode=PS
  Three-Phase V-I Measurement : powerlib/Measurements/Three-Phase V-I Measurement  VoltageMeasurement=phase-to-ground  SetLabelV=off  LabelV=Vabc  Vpu=off  VpuLL=off  CurrentMeasurement=yes  SetLabelI=off  LabelI=Iabc  Ipu=off  Pbase=100e6  Vbase=500e3  OutputType=Complex  PhasorSimulation=on  PSBequivalent=0
      settings: SourceProductName=Simscape Electrical
  A : PMIOPort  Side=Left
  a : PMIOPort  Port=2  Side=Right
  B : PMIOPort  Port=3  Side=Left
  b : PMIOPort  Port=4  Side=Right
  C : PMIOPort  Port=5  Side=Left
  c : PMIOPort  Port=6  Side=Right
  P : Outport
  Q : Outport  Port=2
  wires:
  Three-Phase V-I Measurement/2 -> "Power (3ph, Phasor)"/2
  Three-Phase V-I Measurement/1 -> "Power (3ph, Phasor)"/1
  "Power (3ph, Phasor)"/1 -> P/1
  "Power (3ph, Phasor)"/2 -> Q/1
  connections:
  Three-Phase V-I Measurement/RConn1 -- a/RConn1
  b/RConn1 -- Three-Phase V-I Measurement/RConn2
  A/RConn1 -- Three-Phase V-I Measurement/LConn1
  Three-Phase V-I Measurement/LConn2 -- B/RConn1
  c/RConn1 -- Three-Phase V-I Measurement/RConn3
  C/RConn1 -- Three-Phase V-I Measurement/LConn3

== system tennode_3/DER_Site_3/DER3_BESS/Charge Limits/Overcharge Check ==
  SOC (%) : Inport
  Pin : Inport  Port=2
  Qin : Inport  Port=3
  Backlash : Backlash  BacklashWidth=1e-3  InitialOutput=Initial_kWh_pc  ZeroCross=off
  Compare To Constant : simulink/Logic and Bit Operations/Compare To Constant  relop=>  const=UpChrgLim  OutDataTypeStr=boolean
  Compare To Zero : simulink/Logic and Bit Operations/Compare To Zero  relop=<=  OutDataTypeStr=boolean
  Constant : Constant  Value=0
  Constant1 : Constant  Value=0
  Logical Operator : Logic  AllPortsSameDT=off  OutDataTypeStr=boolean
  Switch : Switch  Criteria=u2 ~= 0
  Switch1 : Switch  Criteria=u2 ~= 0
  Pout : Outport
  Qout : Outport  Port=2
  wires:
  Compare To Constant/1 -> Logical Operator/1
  Logical Operator/1 -> Switch1/2, Switch/2
  Constant/1 -> Switch/1
  SOC (%)/1 -> Backlash/1
  Pin/1 -> Compare To Zero/1, Switch/3
  Switch/1 -> Pout/1
  Compare To Zero/1 -> Logical Operator/2
  Qin/1 -> Switch1/3
  Constant1/1 -> Switch1/1
  Switch1/1 -> Qout/1
  Backlash/1 -> Compare To Constant/1

== system tennode_3/DER_Site_3/DER3_BESS/Charge Limits/Undercharge Check ==
  SOC (%) : Inport
  Pin : Inport  Port=2
  Qin : Inport  Port=3
  Backlash : Backlash  BacklashWidth=1e-3  InitialOutput=Initial_kWh_pc  ZeroCross=off
  Compare To Constant1 : simulink/Logic and Bit Operations/Compare To Constant  relop=<  const=LowChrgLim  OutDataTypeStr=boolean
  Compare To Zero : simulink/Logic and Bit Operations/Compare To Zero  relop=>  OutDataTypeStr=boolean
  Constant{,1..3} (4 alike) : Constant  Value=0
  Constant4 : Constant  Value=autoRecharge
  IC : InitialCondition  Value=RechargeSOC
  Logical Operator : Logic  AllPortsSameDT=off  OutDataTypeStr=boolean
  Relay : Relay  OnSwitchValue=RechargeSOC  OffSwitchValue=LowChrgLim  OnOutputValue=0  OffOutputValue=-Precharge/100*Pnom
  Switch{,1..4} (5 alike) : Switch  Criteria=u2 ~= 0
  Pout : Outport
  Qout : Outport  Port=2
  wires:
  Compare To Zero/1 -> Logical Operator/2
  Pin/1 -> Switch/3, Compare To Zero/1
  SOC (%)/1 -> Backlash/1
  Constant/1 -> Switch/1
  Logical Operator/1 -> Switch/2, Switch1/2
  Compare To Constant1/1 -> Logical Operator/1
  Constant1/1 -> Switch1/1
  Qin/1 -> Switch1/3
  Backlash/1 -> IC/1, Compare To Constant1/1
  Switch4/1 -> Switch2/1, Switch2/2, Switch3/2
  IC/1 -> Relay/1
  Switch/1 -> Switch2/3
  Switch2/1 -> Pout/1
  Switch3/1 -> Qout/1
  Switch1/1 -> Switch3/3
  Constant2/1 -> Switch3/1
  Relay/1 -> Switch4/1
  Constant3/1 -> Switch4/3
  Constant4/1 -> Switch4/2
